simulink model "traffic_light"  (R2024b)
settings: Solver=FixedStepDiscrete  StartTime=0.0  StopTime=10.0  FixedStep=1e-3  RelTol=1e-3  EnableMultiTasking=on
libraries: arduinolib x4
settings Model: ExtModeTrigDuration=2  Creator=Ahmad  LastModifiedBy=Ahmad
settings SolverCC: AutoInsertRateTranBlk=on
settings OptimizationCC: EnhancedBackFolding=on  PassReuseOutputArgsAs=Individual arguments  ZeroExternalMemoryAtStartup=off  ZeroInternalMemoryAtStartup=off  MaxStackSize=64  OptimizeBlockOrder=speed  DifferentSizesBufferReuse=on  OptimizationCustomize=off  EfficientTunableParamExpr=on
settings DebuggingCC: ParameterTunabilityLossMsg=error
settings HardwareCC: ProdBitPerInt=16  ProdBitPerPointer=16  ProdBitPerSizeT=16  ProdBitPerPtrDiffT=16  ProdLargestAtomicFloat=None  ProdWordSize=8  ProdHWDeviceType=Atmel->AVR
settings SFSimCC: MATLABDynamicMemAlloc=off
settings RTWCC: Description=Embedded Coder  SystemTargetFile=ert.tlc  HardwareBoard=Arduino Uno  TemplateMakefile=ert_default_tmf  Toolchain=Arduino AVR  BuildConfiguration=Faster Runs
settings CodeAppCC: ForceParamTrailComments=on  IgnoreCustomStorageClasses=off  OperatorAnnotations=on  SimulinkDataObjDesc=on  SFDataObjDesc=on  InsertBlockDesc=on
settings ERTTargetCC: SupportContinuousTime=on  SupportVariableSizeSignals=on  ExtModeTransport=3  ExtModeStaticAlloc=on  ExtModeAutomaticAllocSize=off  ExtModeStaticAllocSize=250  ExtModeMexFile=ext_xcp  ExtModeIntrfLevel=Level2 - Open  InlinedParameterPlacement=Hierarchical

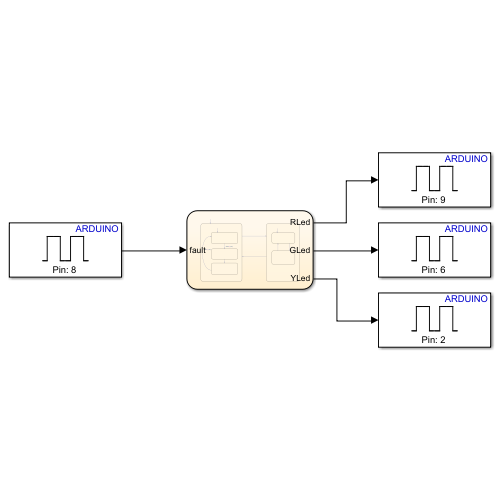
[thumbnail: Simulink's stored preview of the top-level diagram]
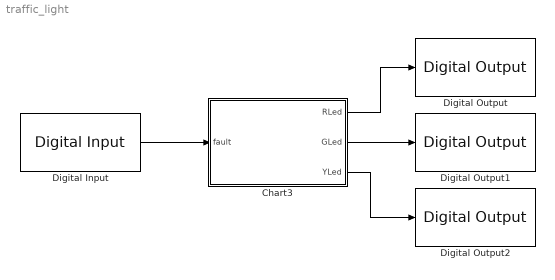
== system traffic_light ==
  Chart3 : Stateflow chart  TreatAsAtomicUnit=on
  Digital Input : arduinolib/Digital Input  pinNumber=8  mode=Input Pullup  Direction=input  SampleTime=0.1  blockPlatform=arduino
  Digital Output : arduinolib/Digital Output  pinNumber=9  Direction=output  blockPlatform=arduino
  Digital Output1 : arduinolib/Digital Output  pinNumber=6  Direction=output  blockPlatform=arduino
  Digital Output2 : arduinolib/Digital Output  pinNumber=2  Direction=output  blockPlatform=arduino
  wires:
  Chart3/1(RLed) -> Digital Output/1
  Chart3/2(GLed) -> Digital Output1/1
  Chart3/3(YLed) -> Digital Output2/1
  Digital Input/1 -> Chart3/1(fault)

== stateflow chart traffic_light/Chart3 ==
  state NormalMode
    state Stop
      entry:
      RLed=1;
      exit:
      RLed=0;
    note: after ( 1 , sec )
    note: after ( 1 , sec )
    state Go
      entry:
      GLed=1;
      exit:
      GLed=0;
    state PTS
      entry:
      YLed=1;
      exit:
      YLed=0;
    (default) -> Stop
    PTS -> Stop
    Stop -> Go
    Go -> PTS : after(1,sec)
  state FaultMode
    state ON
      entry:
      RLed=1;
    state OFF
      entry:
      RLed=0;
    (default) -> ON
    OFF -> ON : after(1,sec)
    ON -> OFF : after(1,sec)
  (default) -> NormalMode
  NormalMode -> FaultMode : [fault==1]
  FaultMode -> NormalMode : [fault==0]
  data: fault input; RLed output; GLed output; YLed output
